simulink model "MPC"  (R2025b)
settings: Solver=ode14x  StartTime=0.0  StopTime=10.0  FixedStep=Ts_local  RelTol=1e-3
values from neighbouring files (symbols this model uses):
  Ts_ctrl = 0.1    [ctrlSys.sldd]
undefined symbols (not defined in the file or in its folder): v_lb, v_ub
libraries: mpclib x1
settings Model: DataDictionary=ctrlSys.sldd  Creator=mercer  LastModifiedBy=mercer

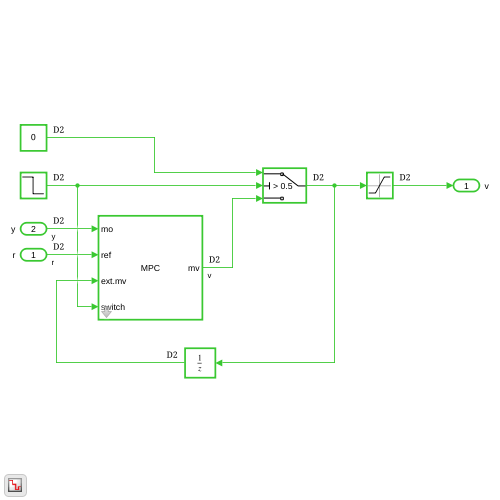
[thumbnail: Simulink's stored preview of the top-level diagram]
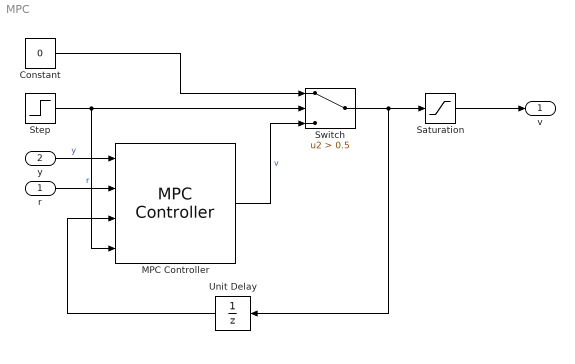
== system MPC ==
  r : Inport  PortDimensions=3
  y : Inport  Port=2  PortDimensions=3
  Constant : Constant  Value=0  SampleTime=Ts_ctrl
  MPC Controller : mpclib/MPC Controller  SCDEnableBlockLinearizationSpecification=on  mpcobj=mpcobj  is_multiple=0  enable_value=0  return_u0=off  updateMPCinCallerWorkspace=on  md_inport=off  mv_inport=on  uref_inport=off  return_cost=off  return_mvseq=off  return_qpstatus=off  return_xseq=off  return_state=off  return_ovseq=off  state_inport=off  umin_inport=off  umax_inport=off  ymin_inport=off  ymax_inport=off  cc_inport=off  ywt_inport=off  uwt_inport=off  duwt_inport=off  rhoeps_inport=off  pm_inport=off  MaximumP=10  HorizonChoice=FixedHorizon  n_ts=0.02  n_p=40  n_mv=3  n_md=0  n_ud=0  n_mo=3  n_uo=0  BlockDataType=double  SampleTimeInherited=off  switch_inport=on
  Saturation : Saturate  UpperLimit=v_ub  LowerLimit=v_lb
  Step : Step  Time=0.5  Before=1  After=0  SampleTime=Ts_ctrl
  Switch : Switch  Criteria=u2 > Threshold  Threshold=0.5  SaturateOnIntegerOverflow=off  InputSameDT=off
  Unit Delay : UnitDelay  SampleTime=-1  HasFrameUpgradeWarning=on
  v : Outport
  wires:
  r/1 -> MPC Controller/2  "r"
  y/1 -> MPC Controller/1  "y"
  Saturation/1 -> v/1
  Switch/1 -> Unit Delay/1, Saturation/1
  MPC Controller/1 -> Switch/3  "v"
  Step/1 -> MPC Controller/4, Switch/2
  Constant/1 -> Switch/1
  Unit Delay/1 -> MPC Controller/3
